simulink model "adaptive"  (R2021a)
settings: Solver=VariableStepAuto  StartTime=0.0  StopTime=100  FixedStep=0.001  RelTol=1e-3
values from neighbouring files (symbols this model uses):
  K_th = eye(3)    [params.m]
undefined symbols (not defined in the file or in its folder): robot
settings Model: Creator=antoninoparisi  LastModifiedBy=antoninoparisi

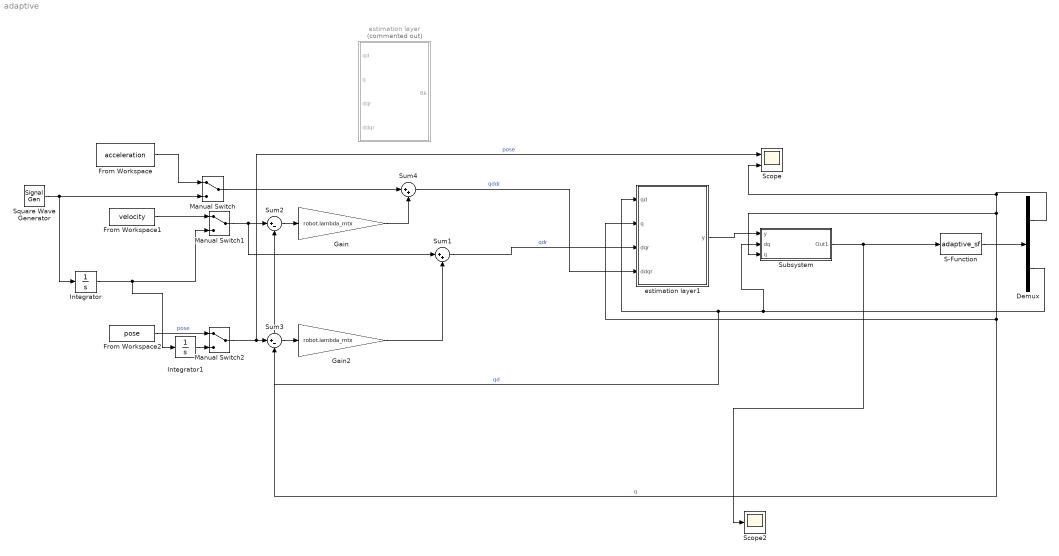
== system adaptive ==
  Demux : Demux  Outputs=2
  From Workspace : FromWorkspace  VariableName=acceleration
  From Workspace1 : FromWorkspace  VariableName=velocity
  From Workspace2 : FromWorkspace  VariableName=pose
  Gain : Gain  Gain=robot.lambda_mtx
  Gain2 : Gain  Gain=robot.lambda_mtx
  Integrator : Integrator
  Integrator1 : Integrator
  Manual Switch : ManualSwitch
  Manual Switch1 : ManualSwitch
  Manual Switch2 : ManualSwitch
  S-Function : S-Function  FunctionName=adaptive_sf  Parameters=robot  SFunctionDeploymentMode=off  EnableBusSupport=off
  Scope : Scope  NumInputPorts=2
  Scope2 : Scope
  Square Wave Generator : SignalGenerator  WaveForm=square  Units=rad/sec
  Subsystem : Subsystem
  Sum1 : Sum  Inputs=|++
  Sum2 : Sum  Inputs=|+-
  Sum3 : Sum  Inputs=|+-
  Sum4 : Sum  Inputs=|++
  estimation layer : Subsystem  Commented=on
  estimation layer1 : Subsystem
  wires:
  Sum2/1 -> Gain/1
  Sum3/1 -> Gain2/1
  Manual Switch/1 -> Sum4/1
  Gain/1 -> Sum4/2
  Manual Switch1/1 -> Sum1/1, Sum2/1
  Manual Switch2/1 -> Scope/1, Sum3/1  "pose"
  Gain2/1 -> Sum1/2
  S-Function/1 -> Demux/1
  Demux/2 -> Subsystem/2(dq), estimation layer1/1(qd), Sum2/2  "qd"
  Demux/1 -> Scope/2, Subsystem/3(q), estimation layer1/2(q), Sum3/2  "q"
  Sum4/1 -> estimation layer1/4(ddqr)  "qddr"
  Sum1/1 -> estimation layer1/3(dqr)  "qdr"
  Subsystem/1(Out1) -> Scope2/1, S-Function/1
  estimation layer1/1(y) -> Subsystem/1(y)
  From Workspace/1 -> Manual Switch/1
  From Workspace1/1 -> Manual Switch1/1
  From Workspace2/1 -> Manual Switch2/1  "pose"
  Square Wave Generator/1 -> Manual Switch/2, Integrator/1
  Integrator/1 -> Integrator1/1, Manual Switch1/2
  Integrator1/1 -> Manual Switch2/2

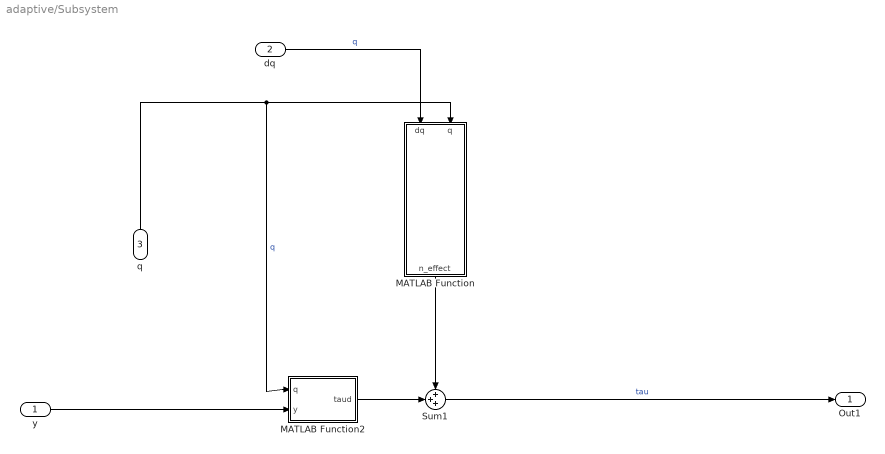
== system adaptive/Subsystem ==
  y : Inport
  dq : Inport  Port=2
  q : Inport  Port=3
  MATLAB Function : MATLAB Function  TreatAsAtomicUnit=on
  MATLAB Function2 : MATLAB Function  TreatAsAtomicUnit=on
  Sum1 : Sum  Inputs=+++
  Out1 : Outport
  wires:
  MATLAB Function/1(n_effect) -> Sum1/1
  MATLAB Function2/1(taud) -> Sum1/2
  q/1 -> MATLAB Function/2(q), MATLAB Function2/1(q)  "q"
  y/1 -> MATLAB Function2/2(y)
  dq/1 -> MATLAB Function/1(dq)  "q"
  Sum1/1 -> Out1/1  "tau"

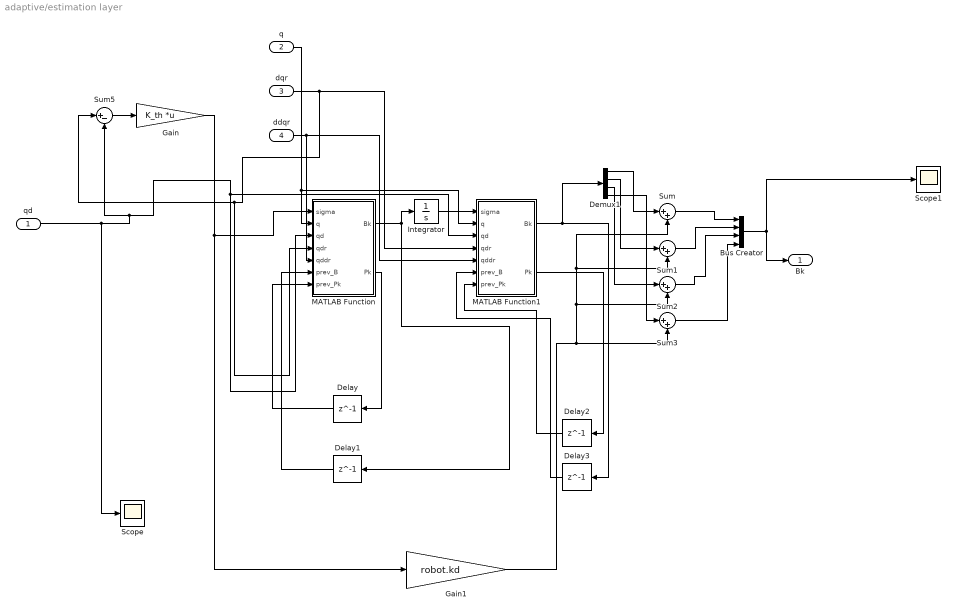
== system adaptive/estimation layer ==
  qd : Inport
  q : Inport  Port=2
  dqr : Inport  Port=3
  ddqr : Inport  Port=4
  Bus Creator : BusCreator  Inputs=4
  Delay{,1..3} (4 alike) : Delay  DelayLength=1
  Demux1 : Demux
  Gain : Gain  Gain=K_th  Multiplication=Matrix(K*u) (u vector)
  Gain1 : Gain  Gain=robot.kd
  Integrator : Integrator
  MATLAB Function : MATLAB Function  TreatAsAtomicUnit=on
  MATLAB Function1 : MATLAB Function  TreatAsAtomicUnit=on
  Scope : Scope
  Scope1 : Scope
  Sum{,1..3} (4 alike) : Sum  Inputs=|++
  Sum5 : Sum  Inputs=|+-
  Bk : Outport  PortDimensions=4
  wires:
  Integrator/1 -> MATLAB Function1/1(sigma)
  MATLAB Function/1(Bk) -> Delay1/1, Integrator/1
  MATLAB Function1/2(Pk) -> Delay2/1
  MATLAB Function/2(Pk) -> Delay/1
  Gain/1 -> Gain1/1, MATLAB Function/1(sigma)
  qd/1 -> MATLAB Function/3(qd), MATLAB Function1/3(qd), Sum5/2, Scope/1
  Gain1/1 -> Sum3/2, Sum2/2, Sum/2, Sum1/2
  q/1 -> MATLAB Function/2(q), MATLAB Function1/2(q)
  dqr/1 -> Sum5/1, MATLAB Function/4(qdr), MATLAB Function1/4(qdr)
  ddqr/1 -> MATLAB Function/5(qddr), MATLAB Function1/5(qddr)
  Sum5/1 -> Gain/1
  Delay/1 -> MATLAB Function/7(prev_Pk)
  Delay1/1 -> MATLAB Function/6(prev_B)
  Delay2/1 -> MATLAB Function1/7(prev_Pk)
  Delay3/1 -> MATLAB Function1/6(prev_B)
  Bus Creator/1 -> Bk/1, Scope1/1
  Sum/1 -> Bus Creator/1
  Sum1/1 -> Bus Creator/2
  Sum2/1 -> Bus Creator/3
  Sum3/1 -> Bus Creator/4
  Demux1/1 -> Sum/1
  Demux1/2 -> Sum1/1
  Demux1/3 -> Sum2/1
  Demux1/4 -> Sum3/1
  MATLAB Function1/1(Bk) -> Demux1/1, Delay3/1

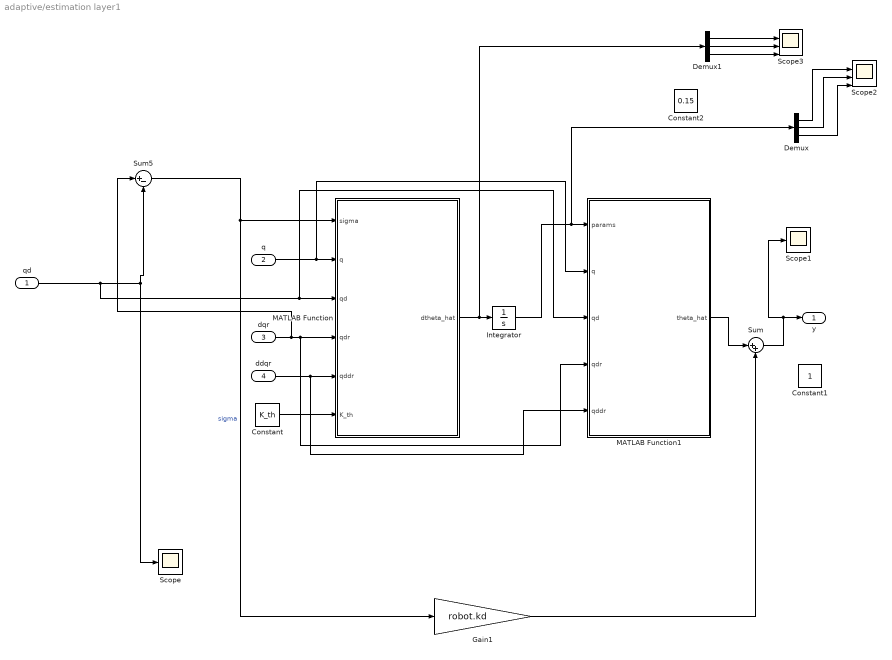
== system adaptive/estimation layer1 ==
  qd : Inport
  q : Inport  Port=2
  dqr : Inport  Port=3
  ddqr : Inport  Port=4
  Constant : Constant  Value=K_th
  Constant1 : Constant
  Constant2 : Constant  Value=0.15
  Demux : Demux  Outputs=3
  Demux1 : Demux  Outputs=3
  Gain1 : Gain  Gain=robot.kd
  Integrator : Integrator
  MATLAB Function : MATLAB Function  TreatAsAtomicUnit=on
  MATLAB Function1 : MATLAB Function  TreatAsAtomicUnit=on
  Scope : Scope
  Scope1 : Scope
  Scope2 : Scope  NumInputPorts=4
  Scope3 : Scope  NumInputPorts=4
  Sum : Sum  Inputs=|++
  Sum5 : Sum  Inputs=|+-
  y : Outport
  wires:
  Sum5/1 -> Gain1/1, MATLAB Function/1(sigma)  "sigma"
  qd/1 -> MATLAB Function1/3(qd), MATLAB Function/3(qd), Sum5/2, Scope/1
  q/1 -> MATLAB Function1/2(q), MATLAB Function/2(q)
  dqr/1 -> Sum5/1, MATLAB Function1/4(qdr), MATLAB Function/4(qdr)
  ddqr/1 -> MATLAB Function1/5(qddr), MATLAB Function/5(qddr)
  Constant/1 -> MATLAB Function/6(K_th)
  Integrator/1 -> Demux/1, MATLAB Function1/1(params)
  Gain1/1 -> Sum/2
  MATLAB Function1/1(theta_hat) -> Sum/1
  Sum/1 -> y/1, Scope1/1
  Demux/1 -> Scope2/2
  Demux/2 -> Scope2/3
  Demux/3 -> Scope2/4
  Demux1/1 -> Scope3/2
  Demux1/3 -> Scope3/4
  Demux1/2 -> Scope3/3
  MATLAB Function/1(dtheta_hat) -> Demux1/1, Integrator/1

== matlab function adaptive/estimation layer/MATLAB Function1 ==
  data: sigma input; q input; qd input; qdr input; qddr input; Bk output size=4; prev_B input; prev_Pk input; Pk output
function [Bk,Pk] = Y_th(sigma,q,qd,qdr,qddr, prev_B, prev_Pk)

% 

if(sum(prev_Pk(:)==0) == 16)
    prev_Pk = diag(diag(prev_Pk+1));
end

lambda = 1;
X = [q,qd,qdr,qddr];

K = [prev_Pk*X'];
Bk = prev_B;
e = [sigma - X*Bk];    

Pk = 1/lambda*(prev_Pk - (prev_Pk*X'*X*prev_Pk)/(lambda + X*prev_Pk*X'));

K = Pk*X';
e = sigma - X*Bk;
Bk = Bk + (K'*e);
% Bk = Bk*[1 1 1 1]';    
end

== matlab function adaptive/estimation layer/MATLAB Function ==
  data: sigma input; q input; qd input; qdr input; qddr input; Bk output size=4; prev_B input; Pk output; prev_Pk input
function [Bk,Pk] = Y_th(sigma,q,qd,qdr,qddr, prev_B, prev_Pk)


if(sum(prev_Pk(:)==0) == 16)
    prev_Pk = diag(diag(prev_Pk+1));
end

% 
lambda = 1;
X = [q,qd,qdr,qddr];

K = [prev_Pk*X'];
Bk = prev_B;
e = [sigma - X*Bk];    

Pk = 1/lambda*(prev_Pk - (prev_Pk*X'*X*prev_Pk)/(lambda + X*prev_Pk*X'));

K = Pk*X';
e = sigma - X*Bk;
Bk = Bk + (K*e);
% Bk = Bk*[1 1 1 1]';    
end

== matlab function adaptive/estimation layer1/MATLAB Function ==
  data: sigma input; dtheta_hat output; q input; qd input; qdr input; qddr input; K_th input
function dtheta_hat = fcn(sigma,q,qd,qdr,qddr, K_th)

    Y = [qddr,qdr,sin(q)]';
    dtheta_hat = pinv(K_th)*Y*sigma(1);

== matlab function adaptive/estimation layer1/MATLAB Function1 ==
  data: params input; theta_hat output; q input; qd input; qdr input; qddr input
function theta_hat = fcn(params,q,qd,qdr,qddr)

    Y = [qddr,qdr,sin(q)];
    theta_hat = Y*params;

== matlab function adaptive/Subsystem/MATLAB Function ==
  data: dq input; q input; n_effect output
function n_effect = n(dq, q)

n_effect = C_Lagrangian(q, dq)*dq + G_Lagrangian(q);

== matlab function adaptive/Subsystem/MATLAB Function2 ==
  data: q input; taud output; y input
function taud = B(q, y)

taud = B_Lagrangian(q)*y;
